simulink model "simpleStateflowModel2"  (R2020b)
settings: Solver=VariableStepAuto  StartTime=0.0  StopTime=10.0  RelTol=1e-3
settings Model: Creator=aarrieta  LastModifiedBy=aarrieta

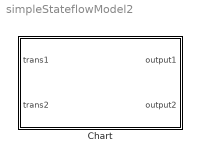
== system simpleStateflowModel2 ==
  Chart : Stateflow chart  TreatAsAtomicUnit=on

== stateflow chart simpleStateflowModel2/Chart ==
  state State1
    entry:
    output1 = 5;
  state State2
    entry:
    output2 = 3;
  state State3
    entry:
    output1 = 3;
  (default) -> State1
  State1 -> State2 : [trans1 == 5]
  State2 -> State1 [order 1] : [trans2 <0]
  State3 -> State1 : [trans2 == 5]
  State2 -> State3 [order 2] : [after(5,msec)]
  data: trans1 input; trans2 input; output1 output; output2 output
